simulink model "RCAM_Aircraft"  (R2026a)
settings: Solver=VariableStepAuto  StopTime=250
values from neighbouring files (symbols this model uses):
  UStar = ZStar(10:14)    [TrimRCAM.m]    (also in trim_values_straight_level.mat = [-6.52622401577e-07 -0.178004826689 -2.27879515584e-06 0.082; validateTrimPoint.m = temp.UStar)
  XStar = ZStar(1:9)    [TrimRCAM.m]    (also in trim_values_straight_level.mat = [84.990495021 1.44774322188e-06 1.2711190394 -3.00658269346e; validateTrimPoint.m = temp.XStar)
undefined symbols (not defined in the file or in its folder): RCAM_Model_D
settings Model: Creator=nuris  LastModifiedBy=nuris

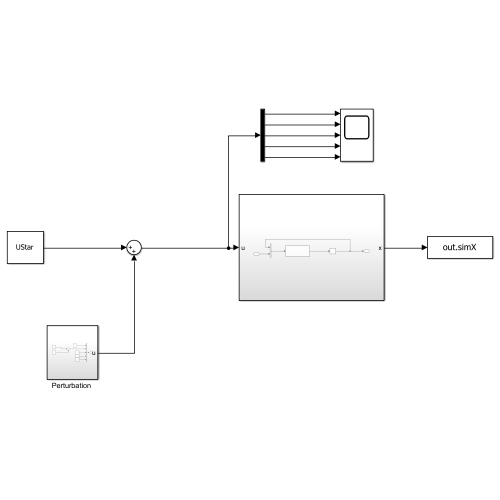
[thumbnail: Simulink's stored preview of the top-level diagram]
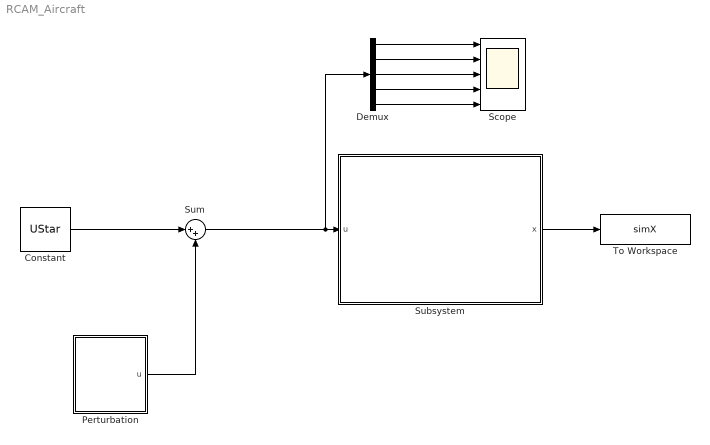
== system RCAM_Aircraft ==
  Constant : Constant  Value=UStar
  Demux : Demux  Outputs=5
  "Perturbation " : Subsystem
  Scope : Scope  NumInputPorts=5
      settings: ActiveDisplayYMinimum=-0.42365801002622172  ActiveDisplayYMaximum=0.034708988428694743
  Subsystem : Subsystem
  Sum : Sum  Inputs=|++
  To Workspace : ToWorkspace  VariableName=simX  SaveFormat=Structure With Time  SampleTime=-1
  wires:
  Subsystem/1(x) -> To Workspace/1
  Demux/5 -> Scope/5
  Demux/4 -> Scope/4
  Demux/3 -> Scope/3
  Demux/2 -> Scope/2
  Demux/1 -> Scope/1
  Constant/1 -> Sum/1
  "Perturbation "/1(u) -> Sum/2
  Sum/1 -> Demux/1, Subsystem/1(u)

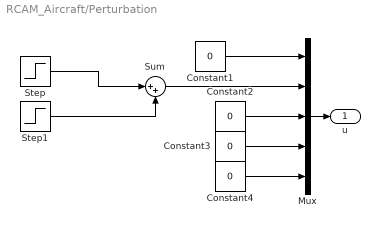
== system RCAM_Aircraft/Perturbation  ==
  Constant{1..4} (4 alike) : Constant  Value=0
  Mux : Mux  Inputs=5
  Step : Step  Time=5  FinalValue=5*pi/180  SampleTime=0
  Step1 : Step  Time=6  FinalValue=-5*pi/180  SampleTime=0
  Sum : Sum  Inputs=|++
  u : Outport
  wires:
  Constant4/1 -> Mux/5
  Constant1/1 -> Mux/1
  Constant3/1 -> Mux/4
  Constant2/1 -> Mux/3
  Mux/1 -> u/1
  Step/1 -> Sum/1
  Step1/1 -> Sum/2
  Sum/1 -> Mux/2

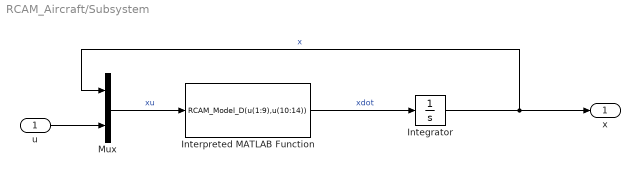
== system RCAM_Aircraft/Subsystem ==
  u : Inport
  Integrator : Integrator  InitialCondition=XStar
  Interpreted MATLAB Function : MATLABFcn  MATLABFcn=RCAM_Model_D(u(1:9),u(10:14))
  Mux : Mux  Inputs=2
  x : Outport
  wires:
  Interpreted MATLAB Function/1 -> Integrator/1  "xdot"
  Integrator/1 -> x/1, Mux/1  "x"
  u/1 -> Mux/2
  Mux/1 -> Interpreted MATLAB Function/1  "xu"
